simulink model "TrackingTest"  (R2013a)
settings: Solver=ode45  StartTime=0.0  StopTime=10  MaxStep=0.00001  RelTol=1e-10
values from neighbouring files (symbols this model uses):
  command_rate = 500    [RunTrackingTest.m]
  measurement_delay = 1    [RunTrackingTest.m]
  measurement_rate = 10    [RunTrackingTest.m]
  measurement_variance = 0.000000001    (= 1e-09)    [RunTrackingTest.m]
  position_time_constant = 1000    [RunTrackingTest.m]
settings Model: Creator=ptm29415  LastModifiedBy=ptm29415

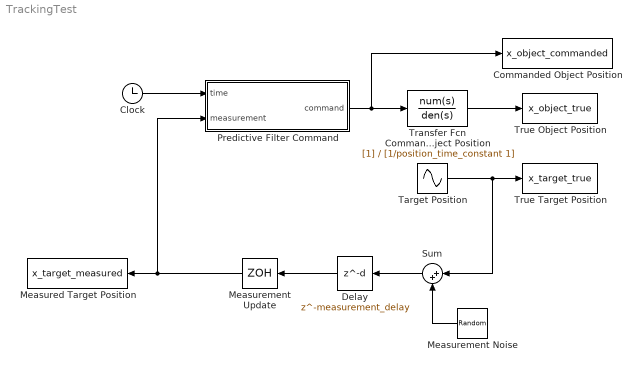
== system TrackingTest ==
  Clock : Clock
  Commanded Object Position : ToWorkspace  VariableName=x_object_commanded  SampleTime=-1  SaveFormat=Timeseries
  Delay : Delay  DelayLength=measurement_delay  InputProcessing=Columns as channels (frame based)  SampleTime=0.00001
  Measured Target Position : ToWorkspace  VariableName=x_target_measured  SampleTime=-1  SaveFormat=Timeseries
  Measurement Noise : RandomNumber  Variance=measurement_variance  SampleTime=0.1
  "Measurement Update " : ZeroOrderHold  SampleTime=1/measurement_rate
  "Predictive Filter Command " : MATLAB Function  TreatAsAtomicUnit=on  SystemSampleTime=1/command_rate
  Sum : Sum  Inputs=|++
  Target Position : Sin  SampleTime=0
  Transfer Fcn Commanded Object Position to True Object Position : TransferFcn  Denominator=[1/position_time_constant 1]
  True Object Position : ToWorkspace  VariableName=x_object_true  SampleTime=-1  SaveFormat=Timeseries
  True Target Position : ToWorkspace  VariableName=x_target_true  SampleTime=-1  SaveFormat=Timeseries
  wires:
  "Measurement Update "/1 -> "Predictive Filter Command "/2(measurement), Measured Target Position/1
  Target Position/1 -> Sum/1, True Target Position/1
  Transfer Fcn Commanded Object Position to True Object Position/1 -> True Object Position/1
  Measurement Noise/1 -> Sum/2
  "Predictive Filter Command "/1(command) -> Commanded Object Position/1, Transfer Fcn Commanded Object Position to True Object Position/1
  Clock/1 -> "Predictive Filter Command "/1(time)
  Sum/1 -> Delay/1
  Delay/1 -> "Measurement Update "/1

== matlab function TrackingTest/Predictive Filter Command  ==
  data: time input; measurement input; command output
function command = fcn(time,measurement)

bin_size = 10;
filter_order = 3;

persistent previous_measurements
persistent previous_timestamps
persistent num_measurements

if isempty(previous_measurements)
    
    % Initialize the empty array of previous measurements
    previous_measurements = zeros(bin_size,1);
    previous_timestamps = zeros(bin_size,1);
    num_measurements = 1;
    
else
    
    if(previous_measurements(end) ~= measurement)
        num_measurements = num_measurements + 1;
        
        % Add the new measurements to the array
        for i = 1:bin_size-1
            previous_measurements(i) = previous_measurements(i+1);
            previous_timestamps(i) = previous_timestamps(i+1);
        end
        previous_measurements(end) = measurement;
        previous_timestamps(end) = time;
    end
    
    
    
end

if (num_measurements > bin_size)
    
    % Fit the data
    P = polyfit(previous_timestamps,previous_measurements,filter_order);
    
    % Calculate the new command (shifted to start at the last recieved measurement)
    command = polyval(P,time) + previous_measurements(end) - polyval(P,previous_timestamps(end));
    
else
    command = measurement;
    
end
